simulink model "main_RI_LIEKF_GNSSOutrage"  (R2023a)
settings: Solver=FixedStepAuto  StartTime=0.0  StopTime=220  FixedStep=0.01  RelTol=1e-3
InitFcn:
  | initNavigation0612_AOA;
values from neighbouring files (symbols this model uses):
  CF_enable = 0    [initNavigation.m]
  dt = 0.01    [initNavigation.m]
  dtDelay = -0.03    [initNavigation.m]
  g0 = 9.795    [initNavigation.m]
  gam0_rad = 0/57.3    (= 0)    [initNavigation.m]
  GNSSoutragetime = 90    [initNavigation.m]
  H_sensor_type = 0    [initNavigation.m]
  KF_enable = 1    [initNavigation.m]
  P0 = diag([1*ones(3,1);0.01*ones(3,1);0.1*ones(3,1);0.001*ones(3,1);0.00001*ones(3,1)])    [initNavigation.m]
  P0_RIEKF = diag([1*ones(3,1);0.01*ones(3,1);0.1*ones(3,1);0.001*ones(3,1);0.00001*ones(3,1);      0.01*ones(3,1);[0;2;2]/57.3;[0.1;0.1;0.1]])^2    [initNavigation.m]
  pd0 = 0    [initNavigation.m]
  pe0 = 0    [initNavigation.m]
  phi0_rad = 0/57.3    (= 0)    [initNavigation.m]
  pn0 = 0    [initNavigation.m]
  psi = -178    [initNavigation.m]
  psi0_rad = 0/57.3    (= 0)    [initNavigation.m]
  state_dim = 24    [initNavigation.m]
  Time = 0:0.01:(size(traindata.AttackAngle,1) - 1)*0.01    [NNLiftCoefficientFit.m]
  vd0 = 0    [initNavigation.m]
  ve0 = 0    [initNavigation.m]
  vn0 = 0    [initNavigation.m]
undefined symbols (not defined in the file or in its folder): DiscIntNeverNeededParam, Discrete, INS_CONST, INS_EXPORT, INS_PARAM, magnitude, p, param, pInitialization, sys
libraries: simulink_extras x94, simulink x82, dspstat3 x70, sharedtransform x60, ctrlSharedLib x36, sharedTrackingLibrary x22, matrix_library x15, FMT_Model_Lib x13, deeplib x8, dspsolvers x4, vrlib x4, aerolibconvert2 x1
(part 21 of 28)

== system main_RI_LIEKF_GNSSOutrage/State estimation/RI EKF_AOA_LSTM/Error State Kalman Filter/bak/Simulink Function - State Transition Jacobian/Cal Phi1 ==
  Rbn : Inport
  vn : Inport  Port=2
  pn : Inport  Port=3
  Constant : Constant  Value=dt
  MATLAB Function1 : MATLAB Function  TreatAsAtomicUnit=on
  Reshape : Reshape  OutputDimensionality=Column vector (2-D)
  Reshape1 : Reshape  OutputDimensionality=Column vector (2-D)
  Phi : Outport
  wires:
  Constant/1 -> MATLAB Function1/4(dt)
  MATLAB Function1/1(Phi) -> Phi/1
  Rbn/1 -> MATLAB Function1/3(Rbn)
  vn/1 -> Reshape/1
  pn/1 -> Reshape1/1
  Reshape/1 -> MATLAB Function1/1(vn)
  Reshape1/1 -> MATLAB Function1/2(pn)

== system main_RI_LIEKF_GNSSOutrage/State estimation/RI EKF_AOA_LSTM/INS propogation/AOA//SA//Vwind update/Subsystem/Subsystem ==
  In1 : Inport
  v : Inport  Port=2
  Asin : Trigonometry  Operator=asin
  Math Function : Math  Operator=magnitude^2
  Product1 : Product
  Reciprocal Sqrt : Sqrt  Operator=rSqrt
  Sum of Elements : Sum  Inputs=+
  beta : Outport
  wires:
  Product1/1 -> Asin/1
  Sum of Elements/1 -> Reciprocal Sqrt/1
  Math Function/1 -> Sum of Elements/1
  Reciprocal Sqrt/1 -> Product1/1
  Asin/1 -> beta/1  "beta"
  In1/1 -> Math Function/1
  v/1 -> Product1/2

== system main_RI_LIEKF_GNSSOutrage/State estimation/RI EKF_AOA_LSTM/INS propogation/AOA//SA//Vwind update/Subsystem/Subsystem1 ==
  gyro_raw : Inport
  elevator_aileron_rudder_deg : Inport  Port=2
  accl_raw : Inport  Port=3
  TAS : Inport  Port=4
  Enable : EnablePort
  Data Type Conversion5 : DataTypeConversion  OutDataTypeStr=single  SaturateOnIntegerOverflow=off  RndMeth=Floor
  Degrees to Radians{,1..5} (6 alike) : simulink_extras/Transformations/Degrees to Radians
  LSTM predict : Subsystem
  LSTM predict1 : Subsystem
  MATLAB Function1 : MATLAB Function  TreatAsAtomicUnit=on
  MATLAB Function3 : MATLAB Function  TreatAsAtomicUnit=on
  MATLAB Function4 : MATLAB Function  Commented=on  TreatAsAtomicUnit=on
  Memory : Memory
  Memory1 : Memory
  Moving Average1 : dspstat3/Moving Average  Method=Sliding window  ForgettingFactorPort=off  SpecifyWindowLength=on  WindowLength=4  OverlapLength=3  AllowArbitraryInputLength=off  ForgettingFactor=0.9  SimulateUsing=Code generation
  Mux : Mux  Inputs=3
  Mux1 : Mux
  Radians to Degrees5 : simulink_extras/Transformations/Radians to Degrees  Commented=on
  Selector : Selector  InputPortWidth=3  IndexOptions=Index vector (dialog)  Indices=[2]  OutputSizes=1
  Selector{1..3,5} (4 alike) : Selector  InputPortWidth=3  IndexOptions=Index vector (dialog)  Indices=[1]  OutputSizes=1
  Selector4 : Selector  InputPortWidth=3  IndexOptions=Index vector (dialog)  Indices=[3]  OutputSizes=1
  Selector6 : Selector  InputPortWidth=3  IndexOptions=Index vector (dialog)  Indices=[3]  OutputSizes=1
  TAS_1 : InportShadow  Port=4
  az : InportShadow  Port=3
  elevator_aileron_rudder_deg_1 : InportShadow  Port=2
  gyro_raw_1 : InportShadow
  AOA_LSTM_rad out : Outport
  SA_LSTM_rad : Outport  Port=2
  wires:
  elevator_aileron_rudder_deg_1/1 -> Selector6/1
  TAS/1 -> Selector2/1
  gyro_raw/1 -> Selector/1
  Degrees to Radians5/1 -> SA_LSTM_rad/1
  Degrees to Radians/1 -> Mux/3
  Selector1/1 -> Degrees to Radians/1
  Memory1/1 -> MATLAB Function3/4(beta)
  MATLAB Function1/1(Cl) -> Data Type Conversion5/1
  accl_raw/1 -> MATLAB Function1/1(axyz)
  Mux/1 -> LSTM predict/1(X), MATLAB Function4/1(u)
  MATLAB Function3/1(Cy) -> Mux1/2
  Selector/1 -> Mux/1
  Selector2/1 -> MATLAB Function1/2(TAS)  "|TAS|"
  LSTM predict1/1(YPred_test_out) -> Degrees to Radians3/1, Degrees to Radians5/1  "LSTM_SA"
  Degrees to Radians3/1 -> Memory1/1
  Degrees to Radians2/1 -> Memory/1
  Degrees to Radians1/1 -> Mux1/3
  az/1 -> MATLAB Function3/1(axyz)
  Selector5/1 -> MATLAB Function3/2(TAS)  "|TAS|"
  TAS_1/1 -> Selector5/1
  LSTM predict/1(YPred_test_out) -> Moving Average1/1, Degrees to Radians4/1
  Degrees to Radians4/1 -> AOA_LSTM_rad out/1
  elevator_aileron_rudder_deg/1 -> Selector1/1
  Memory/1 -> MATLAB Function3/3(alpha), MATLAB Function1/3(alpha)
  Data Type Conversion5/1 -> Mux/2
  Selector6/1 -> Degrees to Radians1/1
  MATLAB Function4/1(CalculatedAttackAngleFiltered) -> Radians to Degrees5/1
  Mux1/1 -> LSTM predict1/1(X)
  Moving Average1/1 -> Degrees to Radians2/1  "LSTM_AOA"
  gyro_raw_1/1 -> Selector3/1, Selector4/1
  Selector3/1 -> Mux1/1
  Selector4/1 -> Mux1/4

== system main_RI_LIEKF_GNSSOutrage/State estimation/RI EKF_AOA_LSTM/INS propogation/AOA//SA//Vwind update/Subsystem/Subsystem2 ==
  In1 : Inport
  v : Inport  Port=2
  Asin : Trigonometry  Operator=asin
  Math Function : Math  Operator=magnitude^2
  Product1 : Product
  Reciprocal Sqrt : Sqrt  Operator=rSqrt
  Sum of Elements : Sum  Inputs=+
  beta : Outport
  wires:
  v/1 -> Product1/2
  In1/1 -> Math Function/1
  Asin/1 -> beta/1  "beta"
  Reciprocal Sqrt/1 -> Product1/1
  Math Function/1 -> Sum of Elements/1
  Sum of Elements/1 -> Reciprocal Sqrt/1
  Product1/1 -> Asin/1

== system main_RI_LIEKF_GNSSOutrage/State estimation/RI EKF_AOA_LSTM/INS propogation/Init_PVQ/Horizontal_attitude/Deal with zero ==
  In1 : Inport
  Add5 : Sum
  Constant1 : Constant  Value=1e-6  OutDataTypeStr=single
  Out1 : Outport
  wires:
  Add5/1 -> Out1/1
  In1/1 -> Add5/1
  Constant1/1 -> Add5/2

== system main_RI_LIEKF_GNSSOutrage/State estimation/RI EKF_AOA_LSTM/INS propogation/gyro bias compensation/error compensation/If Action Subsystem1 ==
  Action Port : ActionPort  ActionPortLabel=if(u1 == 1)
  Constant : Constant
  Data Store Write : DataStoreWrite  DataStoreName=feedback_flag_18dim_RIEKF  IndexOptions=Index vector (dialog)  Indices=1  OutputSizes=1
  wires:
  Constant/1 -> Data Store Write/1

== system main_RI_LIEKF_GNSSOutrage/State estimation/RI EKF_AOA_direct/Error State Kalman Filter/Extended Kalman Filter1/Correct1/IGG_check ==
  Pk/k_1 : Inport
  yMeas : Inport  Port=2
  X : Inport  Port=3
  R : Inport  Port=4
  Abs : Abs  Commented=on  SaturateOnIntegerOverflow=off
  Abs1 : Abs  Commented=on  SaturateOnIntegerOverflow=off
  Add : Sum  Commented=on
  Add1 : Sum  Inputs=+-
  Add2 : Sum  Commented=on
  Constant : Constant  Commented=on  Value=12
  Constant1 : Constant  Commented=on  Value=8
  Constant2 : Constant  Value=25
  Constant3 : Constant  Commented=on  Value=eps
  Constant4 : Constant  Commented=on  Value=15
  Constant6 : Constant  Value=[zeros(6,3),eye(6),zeros(6,6)]  OutDataTypeStr=single
  Divide : Product  Commented=on  Inputs=*/
  Extract Diagonal1 : matrix_library/Extract Diagonal  Commented=on
  MATLAB Function : MATLAB Function  Commented=on  TreatAsAtomicUnit=on
  Product : Product  Inputs=3  Multiplication=Matrix(*)
  Product1 : Product  Multiplication=Matrix(*)
  Product2 : Product
  Scope : Scope  Commented=on
  Sqrt1 : Sqrt  Commented=on
  Transpose : Math  Operator=transpose
  yMeas1 : InportShadow  Port=2
  yMeas_out : Outport
  w : Outport  Port=2
  inno : Outport  Port=3
  wires:
  Constant2/1 -> MATLAB Function/5(zk1)
  Constant/1 -> MATLAB Function/4(zk0)
  Constant4/1 -> MATLAB Function/3(k1)
  Constant1/1 -> MATLAB Function/2(k0)
  yMeas1/1 -> Product2/2
  Constant3/1 -> Add2/2
  Add2/1 -> Divide/2
  Abs1/1 -> Sqrt1/1
  Abs/1 -> MATLAB Function/1(err)
  Sqrt1/1 -> Add2/1
  Add1/1 -> Divide/1, inno/1
  Extract Diagonal1/1 -> Abs1/1
  MATLAB Function/1(w) -> Product2/1, w/1
  Divide/1 -> Scope/1, Abs/1
  Add/1 -> Extract Diagonal1/1  "S"
  Product2/1 -> yMeas_out/1
  Product1/1 -> Add1/2
  X/1 -> Product1/2
  Constant6/1 -> Transpose/1, Product/1, Product1/1
  yMeas/1 -> Add1/1
  Pk/k_1/1 -> Product/2
  R/1 -> Add/2
  Transpose/1 -> Product/3
  Product/1 -> Add/1

== system main_RI_LIEKF_GNSSOutrage/State estimation/RI EKF_AOA_direct/Error State Kalman Filter/Extended Kalman Filter1/Predict/If Action Subsystem ==
  Action Port : ActionPort
  Constant : Constant  Value=0
  Data Store Read : DataStoreRead  DataStoreName=x  IndexOptions=Index vector (dialog)  Indices=1  OutputSizes=1
  Data Store Write : DataStoreWrite  DataStoreName=x  IndexOptions=Index vector (dialog)  Indices=1  OutputSizes=1
  Data Store Write1 : DataStoreWrite  DataStoreName=feedback_flag_18dim  IndexOptions=Index vector (dialog)  Indices=1  OutputSizes=1
  Mux : Mux  Inputs=2
  Selector : Selector  InputPortWidth=18  IndexOptions=Index vector (dialog)  Indices=[16 17 18]  OutputSizes=1
  Zero : Constant  Value=zeros(15,1)  OutDataTypeStr=Inherit: Inherit via back propagation
  wires:
  Constant/1 -> Data Store Write1/1
  Data Store Read/1 -> Selector/1
  Zero/1 -> Mux/1
  Selector/1 -> Mux/2
  Mux/1 -> Data Store Write/1

== system main_RI_LIEKF_GNSSOutrage/State estimation/RI EKF_AOA_direct/Error State Kalman Filter/bak/Simulink Function - State Transition Jacobian/Cal Phi1 ==
  Rbn : Inport
  vn : Inport  Port=2
  pn : Inport  Port=3
  Constant : Constant  Value=dt
  MATLAB Function1 : MATLAB Function  TreatAsAtomicUnit=on
  Reshape : Reshape  OutputDimensionality=Column vector (2-D)
  Reshape1 : Reshape  OutputDimensionality=Column vector (2-D)
  Phi : Outport
  wires:
  Reshape1/1 -> MATLAB Function1/2(pn)
  Reshape/1 -> MATLAB Function1/1(vn)
  pn/1 -> Reshape1/1
  vn/1 -> Reshape/1
  Rbn/1 -> MATLAB Function1/3(Rbn)
  MATLAB Function1/1(Phi) -> Phi/1
  Constant/1 -> MATLAB Function1/4(dt)

== system main_RI_LIEKF_GNSSOutrage/State estimation/RI EKF_AOA_direct/INS propogation/AOA//SA//Vwind update/Subsystem/Subsystem ==
  In1 : Inport
  v : Inport  Port=2
  Asin : Trigonometry  Operator=asin
  Math Function : Math  Operator=magnitude^2
  Product1 : Product
  Reciprocal Sqrt : Sqrt  Operator=rSqrt
  Sum of Elements : Sum  Inputs=+
  beta : Outport
  wires:
  v/1 -> Product1/2
  In1/1 -> Math Function/1
  Asin/1 -> beta/1  "beta"
  Reciprocal Sqrt/1 -> Product1/1
  Math Function/1 -> Sum of Elements/1
  Sum of Elements/1 -> Reciprocal Sqrt/1
  Product1/1 -> Asin/1

== system main_RI_LIEKF_GNSSOutrage/State estimation/RI EKF_AOA_direct/INS propogation/AOA//SA//Vwind update/Subsystem/Subsystem1 ==
  gyro_raw : Inport
  elevator_aileron_rudder_deg : Inport  Port=2
  accl_raw : Inport  Port=3
  TAS : Inport  Port=4
  Enable : EnablePort
  Data Type Conversion5 : DataTypeConversion  OutDataTypeStr=single  SaturateOnIntegerOverflow=off  RndMeth=Floor
  Degrees to Radians{,1..5} (6 alike) : simulink_extras/Transformations/Degrees to Radians
  LSTM predict : Subsystem
  LSTM predict1 : Subsystem
  MATLAB Function1 : MATLAB Function  TreatAsAtomicUnit=on
  MATLAB Function3 : MATLAB Function  TreatAsAtomicUnit=on
  MATLAB Function4 : MATLAB Function  Commented=on  TreatAsAtomicUnit=on
  Memory : Memory
  Memory1 : Memory
  Moving Average : dspstat3/Moving Average  Method=Sliding window  ForgettingFactorPort=off  SpecifyWindowLength=on  WindowLength=4  OverlapLength=3  AllowArbitraryInputLength=off  ForgettingFactor=0.9  SimulateUsing=Code generation
  Moving Average1 : dspstat3/Moving Average  Method=Sliding window  ForgettingFactorPort=off  SpecifyWindowLength=on  WindowLength=4  OverlapLength=3  AllowArbitraryInputLength=off  ForgettingFactor=0.9  SimulateUsing=Code generation
  Mux : Mux  Inputs=3
  Mux1 : Mux
  Radians to Degrees5 : simulink_extras/Transformations/Radians to Degrees  Commented=on
  Selector : Selector  InputPortWidth=3  IndexOptions=Index vector (dialog)  Indices=[2]  OutputSizes=1
  Selector{1..3,5} (4 alike) : Selector  InputPortWidth=3  IndexOptions=Index vector (dialog)  Indices=[1]  OutputSizes=1
  Selector4 : Selector  InputPortWidth=3  IndexOptions=Index vector (dialog)  Indices=[3]  OutputSizes=1
  Selector6 : Selector  InputPortWidth=3  IndexOptions=Index vector (dialog)  Indices=[3]  OutputSizes=1
  TAS_1 : InportShadow  Port=4
  az : InportShadow  Port=3
  elevator_aileron_rudder_deg_1 : InportShadow  Port=2
  gyro_raw_1 : InportShadow
  AOA_LSTM_rad out : Outport
  SA_LSTM_rad : Outport  Port=2
  wires:
  Moving Average1/1 -> Degrees to Radians2/1  "LSTM_AOA"
  Selector4/1 -> Mux1/4
  Mux1/1 -> LSTM predict1/1(X)
  MATLAB Function4/1(CalculatedAttackAngleFiltered) -> Radians to Degrees5/1
  Selector6/1 -> Degrees to Radians1/1
  Data Type Conversion5/1 -> Mux/2
  Selector3/1 -> Mux1/1
  Memory/1 -> MATLAB Function1/3(alpha), MATLAB Function3/3(alpha)
  elevator_aileron_rudder_deg/1 -> Selector1/1
  LSTM predict1/1(YPred_test_out) -> Moving Average/1, Degrees to Radians5/1
  Degrees to Radians4/1 -> AOA_LSTM_rad out/1
  LSTM predict/1(YPred_test_out) -> Degrees to Radians4/1, Moving Average1/1
  TAS_1/1 -> Selector5/1
  Selector5/1 -> MATLAB Function3/2(TAS)  "|TAS|"
  az/1 -> MATLAB Function3/1(axyz)
  Degrees to Radians1/1 -> Mux1/3
  Degrees to Radians2/1 -> Memory/1
  Degrees to Radians3/1 -> Memory1/1
  Moving Average/1 -> Degrees to Radians3/1  "LSTM_SA"
  Selector2/1 -> MATLAB Function1/2(TAS)  "|TAS|"
  Selector/1 -> Mux/1
  MATLAB Function3/1(Cy) -> Mux1/2
  Mux/1 -> MATLAB Function4/1(u), LSTM predict/1(X)
  gyro_raw_1/1 -> Selector4/1, Selector3/1
  accl_raw/1 -> MATLAB Function1/1(axyz)
  MATLAB Function1/1(Cl) -> Data Type Conversion5/1
  Memory1/1 -> MATLAB Function3/4(beta)
  Selector1/1 -> Degrees to Radians/1
  Degrees to Radians/1 -> Mux/3
  Degrees to Radians5/1 -> SA_LSTM_rad/1
  gyro_raw/1 -> Selector/1
  TAS/1 -> Selector2/1
  elevator_aileron_rudder_deg_1/1 -> Selector6/1

== system main_RI_LIEKF_GNSSOutrage/State estimation/RI EKF_AOA_direct/INS propogation/AOA//SA//Vwind update/Subsystem/Subsystem3 ==
  RIEKF_att_Deg : Inport
  vel_NED : Inport  Port=2
  psi_Deg : Inport  Port=3
  Enable : EnablePort
  Add1 : Sum  Inputs=+-
  Add2 : Sum  Inputs=+-
  Asin1 : Trigonometry  Operator=asin
  Atan2 : Trigonometry  Operator=atan2
  Divide1 : Product  Inputs=*/
  Fcn : Fcn  Expr=sqrt(u(1)^2+u(2)^2+u(3)^2)
  Gain : Gain  Gain=-1
  Radians to Degrees{1..4} (4 alike) : simulink_extras/Transformations/Radians to Degrees
  Selector1 : Selector  InputPortWidth=3  IndexOptions=Index vector (dialog)  Indices=[2]  OutputSizes=1
  Selector2 : Selector  InputPortWidth=3  IndexOptions=Index vector (dialog)  Indices=[3]  OutputSizes=1
  Selector3 : Selector  InputPortWidth=3  IndexOptions=Index vector (dialog)  Indices=[1]  OutputSizes=1
  AOA_direct_Deg : Outport
  SA_direct_Deg : Outport  Port=2
  wires:
  RIEKF_att_Deg/1 -> Radians to Degrees2/1
  Radians to Degrees3/1 -> Add1/2  "theta"
  Divide1/1 -> Asin1/1
  Selector2/1 -> Gain/1
  vel_NED/1 -> Selector3/1, Selector1/1, Fcn/1, Selector2/1
  Asin1/1 -> Radians to Degrees3/1
  Fcn/1 -> Divide1/2
  Gain/1 -> Divide1/1
  Add1/1 -> AOA_direct_Deg/1  "AOA_direct"
  Selector1/1 -> Atan2/1
  Selector3/1 -> Atan2/2
  Atan2/1 -> Radians to Degrees1/1
  psi_Deg/1 -> Radians to Degrees4/1
  Radians to Degrees1/1 -> Add2/2  "theta"
  Add2/1 -> SA_direct_Deg/1  "SA_direct"
  Radians to Degrees2/1 -> Add1/1  "theta"
  Radians to Degrees4/1 -> Add2/1  "theta"

== system main_RI_LIEKF_GNSSOutrage/State estimation/RI EKF_AOA_direct/INS propogation/AOA//SA//Vwind update/Subsystem/Subsystem4 ==
  vel_NED : Inport
  Compare To Constant : simulink/Logic and Bit Operations/Compare To Constant  relop=>=  const=10  OutDataTypeStr=boolean
  Math Function : Math  Operator=magnitude^2
  Sqrt : Sqrt
  Sum of Elements : Sum  Inputs=+
  AOA_Estimation_flag : Outport
  wires:
  Sum of Elements/1 -> Sqrt/1
  Sqrt/1 -> Compare To Constant/1
  Compare To Constant/1 -> AOA_Estimation_flag/1
  Math Function/1 -> Sum of Elements/1
  vel_NED/1 -> Math Function/1

== system main_RI_LIEKF_GNSSOutrage/State estimation/RI EKF_AOA_direct/INS propogation/Init_PVQ/Horizontal_attitude/Deal with zero ==
  In1 : Inport
  Add5 : Sum
  Constant1 : Constant  Value=1e-6  OutDataTypeStr=single
  Out1 : Outport
  wires:
  Constant1/1 -> Add5/2
  In1/1 -> Add5/1
  Add5/1 -> Out1/1

== system main_RI_LIEKF_GNSSOutrage/State estimation/RI EKF_AOA_direct/INS propogation/gyro bias compensation/error compensation/If Action Subsystem1 ==
  Action Port : ActionPort  ActionPortLabel=if(u1 == 1)
  Constant : Constant
  Data Store Write : DataStoreWrite  DataStoreName=feedback_flag_18dim_RIEKF  IndexOptions=Index vector (dialog)  Indices=1  OutputSizes=1
  wires:
  Constant/1 -> Data Store Write/1

== system main_RI_LIEKF_GNSSOutrage/State estimation/RI EKF_AOA_ref/Error State Kalman Filter/Extended Kalman Filter1/Correct1/IGG_check ==
  Pk/k_1 : Inport
  yMeas : Inport  Port=2
  X : Inport  Port=3
  R : Inport  Port=4
  Abs : Abs  Commented=on  SaturateOnIntegerOverflow=off
  Abs1 : Abs  Commented=on  SaturateOnIntegerOverflow=off
  Add : Sum  Commented=on
  Add1 : Sum  Inputs=+-
  Add2 : Sum  Commented=on
  Constant : Constant  Commented=on  Value=12
  Constant1 : Constant  Commented=on  Value=8
  Constant2 : Constant  Value=25
  Constant3 : Constant  Commented=on  Value=eps
  Constant4 : Constant  Commented=on  Value=15
  Constant6 : Constant  Value=[zeros(6,3),eye(6),zeros(6,6)]  OutDataTypeStr=single
  Divide : Product  Commented=on  Inputs=*/
  Extract Diagonal1 : matrix_library/Extract Diagonal  Commented=on
  MATLAB Function : MATLAB Function  Commented=on  TreatAsAtomicUnit=on
  Product : Product  Inputs=3  Multiplication=Matrix(*)
  Product1 : Product  Multiplication=Matrix(*)
  Product2 : Product
  Scope : Scope  Commented=on
  Sqrt1 : Sqrt  Commented=on
  Transpose : Math  Operator=transpose
  yMeas1 : InportShadow  Port=2
  yMeas_out : Outport
  w : Outport  Port=2
  inno : Outport  Port=3
  wires:
  Constant2/1 -> MATLAB Function/5(zk1)
  Constant/1 -> MATLAB Function/4(zk0)
  Constant4/1 -> MATLAB Function/3(k1)
  Constant1/1 -> MATLAB Function/2(k0)
  yMeas1/1 -> Product2/2
  Constant3/1 -> Add2/2
  Add2/1 -> Divide/2
  Abs1/1 -> Sqrt1/1
  Abs/1 -> MATLAB Function/1(err)
  Sqrt1/1 -> Add2/1
  Add1/1 -> Divide/1, inno/1
  Extract Diagonal1/1 -> Abs1/1
  MATLAB Function/1(w) -> Product2/1, w/1
  Divide/1 -> Scope/1, Abs/1
  Add/1 -> Extract Diagonal1/1  "S"
  Product2/1 -> yMeas_out/1
  Product1/1 -> Add1/2
  X/1 -> Product1/2
  Constant6/1 -> Transpose/1, Product/1, Product1/1
  yMeas/1 -> Add1/1
  Pk/k_1/1 -> Product/2
  R/1 -> Add/2
  Transpose/1 -> Product/3
  Product/1 -> Add/1

== system main_RI_LIEKF_GNSSOutrage/State estimation/RI EKF_AOA_ref/Error State Kalman Filter/Extended Kalman Filter1/Predict/If Action Subsystem ==
  Action Port : ActionPort
  Constant : Constant  Value=0
  Data Store Read : DataStoreRead  DataStoreName=x  IndexOptions=Index vector (dialog)  Indices=1  OutputSizes=1
  Data Store Write : DataStoreWrite  DataStoreName=x  IndexOptions=Index vector (dialog)  Indices=1  OutputSizes=1
  Data Store Write1 : DataStoreWrite  DataStoreName=feedback_flag_18dim  IndexOptions=Index vector (dialog)  Indices=1  OutputSizes=1
  Mux : Mux  Inputs=2
  Selector : Selector  InputPortWidth=18  IndexOptions=Index vector (dialog)  Indices=[16 17 18]  OutputSizes=1
  Zero : Constant  Value=zeros(15,1)  OutDataTypeStr=Inherit: Inherit via back propagation
  wires:
  Constant/1 -> Data Store Write1/1
  Data Store Read/1 -> Selector/1
  Zero/1 -> Mux/1
  Selector/1 -> Mux/2
  Mux/1 -> Data Store Write/1

== system main_RI_LIEKF_GNSSOutrage/State estimation/RI EKF_AOA_ref/Error State Kalman Filter/bak/Simulink Function - State Transition Jacobian/Cal Phi1 ==
  Rbn : Inport
  vn : Inport  Port=2
  pn : Inport  Port=3
  Constant : Constant  Value=dt
  MATLAB Function1 : MATLAB Function  TreatAsAtomicUnit=on
  Reshape : Reshape  OutputDimensionality=Column vector (2-D)
  Reshape1 : Reshape  OutputDimensionality=Column vector (2-D)
  Phi : Outport
  wires:
  Reshape1/1 -> MATLAB Function1/2(pn)
  Reshape/1 -> MATLAB Function1/1(vn)
  pn/1 -> Reshape1/1
  vn/1 -> Reshape/1
  Rbn/1 -> MATLAB Function1/3(Rbn)
  MATLAB Function1/1(Phi) -> Phi/1
  Constant/1 -> MATLAB Function1/4(dt)

== system main_RI_LIEKF_GNSSOutrage/State estimation/RI EKF_AOA_ref/INS propogation/AOA//SA//Vwind update/Subsystem/Subsystem ==
  In1 : Inport
  v : Inport  Port=2
  Asin : Trigonometry  Operator=asin
  Math Function : Math  Operator=magnitude^2
  Product1 : Product
  Reciprocal Sqrt : Sqrt  Operator=rSqrt
  Sum of Elements : Sum  Inputs=+
  beta : Outport
  wires:
  v/1 -> Product1/2
  In1/1 -> Math Function/1
  Asin/1 -> beta/1  "beta"
  Reciprocal Sqrt/1 -> Product1/1
  Math Function/1 -> Sum of Elements/1
  Sum of Elements/1 -> Reciprocal Sqrt/1
  Product1/1 -> Asin/1

== system main_RI_LIEKF_GNSSOutrage/State estimation/RI EKF_AOA_ref/INS propogation/AOA//SA//Vwind update/Subsystem/Subsystem1 ==
  gyro_raw : Inport
  elevator_aileron_rudder_deg : Inport  Port=2
  accl_raw : Inport  Port=3
  TAS : Inport  Port=4
  Enable : EnablePort
  Data Type Conversion5 : DataTypeConversion  OutDataTypeStr=single  SaturateOnIntegerOverflow=off  RndMeth=Floor
  Degrees to Radians{,1..5} (6 alike) : simulink_extras/Transformations/Degrees to Radians
  LSTM predict : Subsystem
  LSTM predict1 : Subsystem
  MATLAB Function1 : MATLAB Function  TreatAsAtomicUnit=on
  MATLAB Function3 : MATLAB Function  TreatAsAtomicUnit=on
  MATLAB Function4 : MATLAB Function  Commented=on  TreatAsAtomicUnit=on
  Memory : Memory
  Memory1 : Memory
  Moving Average1 : dspstat3/Moving Average  Method=Sliding window  ForgettingFactorPort=off  SpecifyWindowLength=on  WindowLength=4  OverlapLength=3  AllowArbitraryInputLength=off  ForgettingFactor=0.9  SimulateUsing=Code generation
  Mux : Mux  Inputs=3
  Mux1 : Mux
  Radians to Degrees5 : simulink_extras/Transformations/Radians to Degrees  Commented=on
  Selector : Selector  InputPortWidth=3  IndexOptions=Index vector (dialog)  Indices=[2]  OutputSizes=1
  Selector{1..3,5} (4 alike) : Selector  InputPortWidth=3  IndexOptions=Index vector (dialog)  Indices=[1]  OutputSizes=1
  Selector4 : Selector  InputPortWidth=3  IndexOptions=Index vector (dialog)  Indices=[3]  OutputSizes=1
  Selector6 : Selector  InputPortWidth=3  IndexOptions=Index vector (dialog)  Indices=[3]  OutputSizes=1
  TAS_1 : InportShadow  Port=4
  az : InportShadow  Port=3
  elevator_aileron_rudder_deg_1 : InportShadow  Port=2
  gyro_raw_1 : InportShadow
  AOA_LSTM_rad out : Outport
  SA_LSTM_rad : Outport  Port=2
  wires:
  Selector4/1 -> Mux1/4
  Selector3/1 -> Mux1/1
  gyro_raw_1/1 -> Selector4/1, Selector3/1
  Moving Average1/1 -> Degrees to Radians2/1  "LSTM_AOA"
  Mux1/1 -> LSTM predict1/1(X)
  MATLAB Function4/1(CalculatedAttackAngleFiltered) -> Radians to Degrees5/1
  Selector6/1 -> Degrees to Radians1/1
  Data Type Conversion5/1 -> Mux/2
  Memory/1 -> MATLAB Function1/3(alpha), MATLAB Function3/3(alpha)
  elevator_aileron_rudder_deg/1 -> Selector1/1
  Degrees to Radians4/1 -> AOA_LSTM_rad out/1
  LSTM predict/1(YPred_test_out) -> Degrees to Radians4/1, Moving Average1/1
  TAS_1/1 -> Selector5/1
  Selector5/1 -> MATLAB Function3/2(TAS)  "|TAS|"
  az/1 -> MATLAB Function3/1(axyz)
  Degrees to Radians1/1 -> Mux1/3
  Degrees to Radians2/1 -> Memory/1
  Degrees to Radians3/1 -> Memory1/1
  LSTM predict1/1(YPred_test_out) -> Degrees to Radians5/1, Degrees to Radians3/1  "LSTM_SA"
  Selector2/1 -> MATLAB Function1/2(TAS)  "|TAS|"
  Selector/1 -> Mux/1
  MATLAB Function3/1(Cy) -> Mux1/2
  Mux/1 -> MATLAB Function4/1(u), LSTM predict/1(X)
  accl_raw/1 -> MATLAB Function1/1(axyz)
  MATLAB Function1/1(Cl) -> Data Type Conversion5/1
  Memory1/1 -> MATLAB Function3/4(beta)
  Selector1/1 -> Degrees to Radians/1
  Degrees to Radians/1 -> Mux/3
  Degrees to Radians5/1 -> SA_LSTM_rad/1
  gyro_raw/1 -> Selector/1
  TAS/1 -> Selector2/1
  elevator_aileron_rudder_deg_1/1 -> Selector6/1

== system main_RI_LIEKF_GNSSOutrage/State estimation/RI EKF_AOA_ref/INS propogation/AOA//SA//Vwind update/Subsystem/Subsystem2 ==
  In1 : Inport
  v : Inport  Port=2
  Asin : Trigonometry  Operator=asin
  Math Function : Math  Operator=magnitude^2
  Product1 : Product
  Reciprocal Sqrt : Sqrt  Operator=rSqrt
  Sum of Elements : Sum  Inputs=+
  beta : Outport
  wires:
  Product1/1 -> Asin/1
  Sum of Elements/1 -> Reciprocal Sqrt/1
  Math Function/1 -> Sum of Elements/1
  Reciprocal Sqrt/1 -> Product1/1
  Asin/1 -> beta/1  "beta"
  In1/1 -> Math Function/1
  v/1 -> Product1/2

== system main_RI_LIEKF_GNSSOutrage/State estimation/RI EKF_AOA_ref/INS propogation/Init_PVQ/Horizontal_attitude/Deal with zero ==
  In1 : Inport
  Add5 : Sum
  Constant1 : Constant  Value=1e-6  OutDataTypeStr=single
  Out1 : Outport
  wires:
  Constant1/1 -> Add5/2
  In1/1 -> Add5/1
  Add5/1 -> Out1/1

== system main_RI_LIEKF_GNSSOutrage/State estimation/RI EKF_AOA_ref/INS propogation/gyro bias compensation/error compensation/If Action Subsystem1 ==
  Action Port : ActionPort  ActionPortLabel=if(u1 == 1)
  Constant : Constant
  Data Store Write : DataStoreWrite  DataStoreName=feedback_flag_18dim_RIEKF  IndexOptions=Index vector (dialog)  Indices=1  OutputSizes=1
  wires:
  Constant/1 -> Data Store Write/1

== system main_RI_LIEKF_GNSSOutrage/State estimation/RI UKF/Error State Kalman Filter/bak/Simulink Function - State Transition Jacobian/Cal Phi1 ==
  Rbn : Inport
  vn : Inport  Port=2
  pn : Inport  Port=3
  Constant : Constant  Value=dt
  MATLAB Function1 : MATLAB Function  TreatAsAtomicUnit=on
  Reshape : Reshape  OutputDimensionality=Column vector (2-D)
  Reshape1 : Reshape  OutputDimensionality=Column vector (2-D)
  Phi : Outport
  wires:
  Constant/1 -> MATLAB Function1/4(dt)
  MATLAB Function1/1(Phi) -> Phi/1
  Rbn/1 -> MATLAB Function1/3(Rbn)
  vn/1 -> Reshape/1
  pn/1 -> Reshape1/1
  Reshape/1 -> MATLAB Function1/1(vn)
  Reshape1/1 -> MATLAB Function1/2(pn)

== system main_RI_LIEKF_GNSSOutrage/State estimation/RI UKF/INS propogation/AOA//SA//Vwind update/Subsystem/Subsystem ==
  In1 : Inport
  v : Inport  Port=2
  Asin : Trigonometry  Operator=asin
  Math Function : Math  Operator=magnitude^2
  Product1 : Product
  Reciprocal Sqrt : Sqrt  Operator=rSqrt
  Sum of Elements : Sum  Inputs=+
  beta : Outport
  wires:
  Product1/1 -> Asin/1
  Sum of Elements/1 -> Reciprocal Sqrt/1
  Math Function/1 -> Sum of Elements/1
  Reciprocal Sqrt/1 -> Product1/1
  Asin/1 -> beta/1  "beta"
  In1/1 -> Math Function/1
  v/1 -> Product1/2

== system main_RI_LIEKF_GNSSOutrage/State estimation/RI UKF/INS propogation/Init_PVQ/Horizontal_attitude/Deal with zero ==
  In1 : Inport
  Add5 : Sum
  Constant1 : Constant  Value=1e-6  OutDataTypeStr=single
  Out1 : Outport
  wires:
  Add5/1 -> Out1/1
  In1/1 -> Add5/1
  Constant1/1 -> Add5/2

== system main_RI_LIEKF_GNSSOutrage/State estimation/RI UKF/INS propogation/gyro bias compensation/error compensation/If Action Subsystem1 ==
  Action Port : ActionPort  ActionPortLabel=if(u1 == 1)
  Constant : Constant
  Data Store Write : DataStoreWrite  DataStoreName=feedback_flag_18dim  IndexOptions=Index vector (dialog)  Indices=1  OutputSizes=1
  wires:
  Constant/1 -> Data Store Write/1

== system main_RI_LIEKF_GNSSOutrage/State estimation/bak1/Error State Kalman Filter/Extended Kalman Filter1/Correct1/IGG_check ==
  Pk/k_1 : Inport
  yMeas : Inport  Port=2
  X : Inport  Port=3
  R : Inport  Port=4
  Abs : Abs  SaturateOnIntegerOverflow=off
  Abs1 : Abs  SaturateOnIntegerOverflow=off
  Add : Sum
  Add1 : Sum  Inputs=+-
  Add2 : Sum
  Constant : Constant  Value=12
  Constant1 : Constant  Value=8
  Constant2 : Constant  Value=25
  Constant3 : Constant  Value=eps
  Constant4 : Constant  Value=15
  Constant6 : Constant  Value=[eye(3),zeros(3,15)]  OutDataTypeStr=single
  Divide : Product  Inputs=*/
  Extract Diagonal1 : matrix_library/Extract Diagonal
  MATLAB Function : MATLAB Function  TreatAsAtomicUnit=on
  Product : Product  Inputs=3  Multiplication=Matrix(*)
  Product1 : Product  Multiplication=Matrix(*)
  Product2 : Product
  Scope : Scope
  Sqrt1 : Sqrt
  Transpose : Math  Operator=transpose
  yMeas1 : InportShadow  Port=2
  yMeas_out : Outport
  w : Outport  Port=2
  wires:
  Constant2/1 -> MATLAB Function/5(zk1)
  Constant/1 -> MATLAB Function/4(zk0)
  Constant4/1 -> MATLAB Function/3(k1)
  Constant1/1 -> MATLAB Function/2(k0)
  yMeas1/1 -> Product2/2
  Constant3/1 -> Add2/2
  Add2/1 -> Divide/2
  Abs1/1 -> Sqrt1/1
  Abs/1 -> MATLAB Function/1(err)
  Sqrt1/1 -> Add2/1
  Add1/1 -> Divide/1
  Extract Diagonal1/1 -> Abs1/1
  MATLAB Function/1(w) -> Product2/1, w/1
  Divide/1 -> Scope/1, Abs/1
  Add/1 -> Extract Diagonal1/1  "S"
  Product2/1 -> yMeas_out/1
  Product1/1 -> Add1/2
  X/1 -> Product1/2
  Constant6/1 -> Transpose/1, Product/1, Product1/1
  yMeas/1 -> Add1/1
  Pk/k_1/1 -> Product/2
  R/1 -> Add/2
  Transpose/1 -> Product/3
  Product/1 -> Add/1

== system main_RI_LIEKF_GNSSOutrage/State estimation/bak1/Error State Kalman Filter/Extended Kalman Filter1/Predict/If Action Subsystem ==
  Action Port : ActionPort
  Constant : Constant  Value=0
  Data Store Read : DataStoreRead  DataStoreName=x  IndexOptions=Index vector (dialog)  Indices=1  OutputSizes=1
  Data Store Write : DataStoreWrite  DataStoreName=x  IndexOptions=Index vector (dialog)  Indices=1  OutputSizes=1
  Data Store Write1 : DataStoreWrite  DataStoreName=feedback_flag_18dim  IndexOptions=Index vector (dialog)  Indices=1  OutputSizes=1
  Mux : Mux  Inputs=2
  Selector : Selector  InputPortWidth=18  IndexOptions=Index vector (dialog)  Indices=[16 17 18]  OutputSizes=1
  Zero : Constant  Value=zeros(15,1)  OutDataTypeStr=Inherit: Inherit via back propagation
  wires:
  Constant/1 -> Data Store Write1/1
  Data Store Read/1 -> Selector/1
  Zero/1 -> Mux/1
  Selector/1 -> Mux/2
  Mux/1 -> Data Store Write/1

== system main_RI_LIEKF_GNSSOutrage/State estimation/bak1/INS propogation/Init_PVQ/Horizontal_attitude/Deal with zero ==
  In1 : Inport
  Add5 : Sum
  Constant1 : Constant  Value=1e-6  OutDataTypeStr=single
  Out1 : Outport
  wires:
  Constant1/1 -> Add5/2
  In1/1 -> Add5/1
  Add5/1 -> Out1/1

== system main_RI_LIEKF_GNSSOutrage/State estimation/bak1/INS propogation/gyro bias compensation/error compensation/If Action Subsystem1 ==
  Action Port : ActionPort
  Constant : Constant
  Data Store Write : DataStoreWrite  DataStoreName=feedback_flag_18dim  IndexOptions=Index vector (dialog)  Indices=1  OutputSizes=1
  wires:
  Constant/1 -> Data Store Write/1

== system main_RI_LIEKF_GNSSOutrage/State estimation/distribute CF/AHRS/AHRS Complementary filter/Complementary Filter/Cross-product ==
  vactor_A : Inport
  vactor_B : Inport  Port=2
  Bus Creator : BusCreator  Inputs=6
  Demux : Demux  Outputs=3
  Demux1 : Demux  Outputs=3
  Fcn : Fcn  Expr=u(2)*u(6)-u(3)*u(5)
  Fcn1 : Fcn  Expr=u(3)*u(4)-u(1)*u(6)
  Fcn2 : Fcn  Expr=u(1)*u(5)-u(2)*u(4)
  Mux2 : Mux  Inputs=3
  vactor_error_A&B : Outport
  wires:
  Demux/1 -> Bus Creator/1
  Demux/2 -> Bus Creator/2
  Demux/3 -> Bus Creator/3
  Demux1/1 -> Bus Creator/4
  Demux1/2 -> Bus Creator/5
  Demux1/3 -> Bus Creator/6
  Bus Creator/1 -> Fcn2/1, Fcn1/1, Fcn/1
  Fcn/1 -> Mux2/1
  Fcn1/1 -> Mux2/2
  Fcn2/1 -> Mux2/3
  vactor_A/1 -> Demux/1
  Mux2/1 -> vactor_error_A&B/1
  vactor_B/1 -> Demux1/1

== system main_RI_LIEKF_GNSSOutrage/State estimation/distribute CF/AHRS/AHRS Complementary filter/Complementary Filter/Normalized ==
  fb : Inport
  Divide : Product  Inputs=*/
  Math Function : Math  Operator=magnitude^2  SignedPower=on
  Sqrt : Sqrt
  Sum of Elements : Sum  Inputs=+
  fb/g : Outport
  wires:
  Math Function/1 -> Sum of Elements/1
  Divide/1 -> fb/g/1
  Sum of Elements/1 -> Sqrt/1
  fb/1 -> Divide/1, Math Function/1
  Sqrt/1 -> Divide/2

== system main_RI_LIEKF_GNSSOutrage/State estimation/distribute CF/AHRS/AHRS Complementary filter/Complementary Filter/Normalized1 ==
  fb_estimatedValue : Inport
  Divide : Product  Inputs=*/
  Math Function : Math  Operator=magnitude^2  SignedPower=on
  Sqrt : Sqrt
  Sum of Elements : Sum  Inputs=+
  fb_estimatedValue_Normalized : Outport
  wires:
  Math Function/1 -> Sum of Elements/1
  Divide/1 -> fb_estimatedValue_Normalized/1
  Sum of Elements/1 -> Sqrt/1
  fb_estimatedValue/1 -> Divide/1, Math Function/1
  Sqrt/1 -> Divide/2

== system main_RI_LIEKF_GNSSOutrage/State estimation/distribute CF/AHRS/AHRS Complementary filter/MagnHeadingCorrect/Subsystem6 ==
  m : Inport
  Add : Sum  Inputs=3
  Demux : Demux  Outputs=3
  Divide : Product  Inputs=*/
  Dot Product : DotProduct  OutDataTypeStr=Inherit: Inherit via internal rule
  Dot Product1 : DotProduct  OutDataTypeStr=Inherit: Inherit via internal rule
  Dot Product2 : DotProduct  OutDataTypeStr=Inherit: Inherit via internal rule
  Sqrt : Sqrt
  Switch : Switch  Criteria=u2 > Threshold  SaturateOnIntegerOverflow=off  InputSameDT=off
  z : Constant  Value=zeros(3,1)  OutDataTypeStr=single
  m/|m| : Outport
  wires:
  Switch/1 -> m/|m|/1
  z/1 -> Switch/3
  Sqrt/1 -> Divide/2, Switch/2
  Dot Product2/1 -> Add/3
  Dot Product/1 -> Add/1
  Dot Product1/1 -> Add/2
  Demux/1 -> Dot Product/2, Dot Product/1
  m/1 -> Demux/1, Divide/1
  Add/1 -> Sqrt/1
  Divide/1 -> Switch/1
  Demux/3 -> Dot Product2/1, Dot Product2/2
  Demux/2 -> Dot Product1/1, Dot Product1/2

== system main_RI_LIEKF_GNSSOutrage/State estimation/distribute CF/AHRS/AHRS Complementary filter/MagnHeadingCorrect/chacheng6 ==
  In1 : Inport
  In2 : Inport  Port=2
  Bus Creator : BusCreator  Inputs=6
  Demux : Demux  Outputs=3
  Demux1 : Demux  Outputs=3
  Fcn : Fcn  Expr=u(2)*u(6)-u(3)*u(5)
  Fcn1 : Fcn  Expr=u(3)*u(4)-u(1)*u(6)
  Fcn2 : Fcn  Expr=u(1)*u(5)-u(2)*u(4)
  Mux2 : Mux  Inputs=3
  Out1 : Outport
  wires:
  In2/1 -> Demux1/1
  Mux2/1 -> Out1/1
  In1/1 -> Demux/1
  Fcn2/1 -> Mux2/3
  Fcn1/1 -> Mux2/2
  Fcn/1 -> Mux2/1
  Bus Creator/1 -> Fcn2/1, Fcn1/1, Fcn/1
  Demux1/3 -> Bus Creator/6
  Demux1/2 -> Bus Creator/5
  Demux1/1 -> Bus Creator/4
  Demux/3 -> Bus Creator/3
  Demux/2 -> Bus Creator/2
  Demux/1 -> Bus Creator/1

== system main_RI_LIEKF_GNSSOutrage/State estimation/distribute CF/AHRS/AHRS Complementary filter/manoeuvrable check/manoeuvrable check ==
  fn : Inport
  eular : Inport  Port=2
  manoeuvrable check : MATLAB Function  TreatAsAtomicUnit=on
  flag : Outport
  wires:
  eular/1 -> manoeuvrable check/2(eular)
  manoeuvrable check/1(flag) -> flag/1
  fn/1 -> manoeuvrable check/1(fn)

== system main_RI_LIEKF_GNSSOutrage/State estimation/distribute CF/AHRS/Init_Q0/Horizontal_attitude/Deal with zero ==
  In1 : Inport
  Add5 : Sum
  Constant1 : Constant  Value=1e-6  OutDataTypeStr=single
  Out1 : Outport
  wires:
  Constant1/1 -> Add5/2
  In1/1 -> Add5/1
  Add5/1 -> Out1/1

== system main_RI_LIEKF_GNSSOutrage/State estimation/distribute CF/Translation_estimate/Rxy_Horizontal_estimation/Rxy_kalman filter2/Vxy kalman filter ==
  Z : Inport
  F : Inport  Port=2
  G : Inport  Port=3
  H : Inport  Port=4
  Q : Inport  Port=5
  R : Inport  Port=6
  X : Inport  Port=7
  P0 : Inport  Port=8
  Enable : Inport  Port=9
  Add1 : Sum
  Delay : Delay  DelayLength=1  InitialConditionSource=Input port
      settings: InputPortMap=u0,p4
  Gain4 : Gain  Gain=0.5
  Math Function : Math  Operator=transpose  SignedPower=on
  kalman : Subsystem
  XOut : Outport
  wires:
  P0/1 -> Delay/2
  Gain4/1 -> Delay/1
  Delay/1 -> kalman/7(P)
  Add1/1 -> Gain4/1
  Math Function/1 -> Add1/2
  Z/1 -> kalman/1(Z)
  F/1 -> kalman/2(F)
  G/1 -> kalman/3(G)
  H/1 -> kalman/4(H)
  Q/1 -> kalman/5(Q)
  R/1 -> kalman/6(R)
  X/1 -> kalman/8(X)
  kalman/1(POut) -> Math Function/1, Add1/1
  kalman/2(XOut) -> XOut/1
  Enable/1 -> kalman/9(Enable)

== system main_RI_LIEKF_GNSSOutrage/State estimation/distribute CF/Translation_estimate/V_Horizontal_estimation/Rxy_kalman filter1/Vxy kalman filter ==
  Z : Inport
  F : Inport  Port=2
  G : Inport  Port=3
  H : Inport  Port=4
  Q : Inport  Port=5
  R : Inport  Port=6
  X : Inport  Port=7
  P0 : Inport  Port=8
  Enable : Inport  Port=9
  Add1 : Sum
  Delay : Delay  DelayLength=1  InitialConditionSource=Input port
      settings: InputPortMap=u0,p4
  Gain4 : Gain  Gain=0.5
  Math Function : Math  Operator=transpose  SignedPower=on
  kalman : Subsystem
  XOut : Outport
  wires:
  Enable/1 -> kalman/9(Enable)
  kalman/2(XOut) -> XOut/1
  kalman/1(POut) -> Add1/1, Math Function/1
  X/1 -> kalman/8(X)
  R/1 -> kalman/6(R)
  Q/1 -> kalman/5(Q)
  H/1 -> kalman/4(H)
  G/1 -> kalman/3(G)
  F/1 -> kalman/2(F)
  Z/1 -> kalman/1(Z)
  Math Function/1 -> Add1/2
  Add1/1 -> Gain4/1
  Delay/1 -> kalman/7(P)
  Gain4/1 -> Delay/1
  P0/1 -> Delay/2

== system main_RI_LIEKF_GNSSOutrage/State estimation/distribute CF/distribute CF/AHRS1/Bus_Constructor/Euler_Angle ==
  att_quat : Inport
  Demux : Demux  Outputs=3
  Quaternion To Euler : FMT_Model_Lib/Quaternion/Quaternion To Euler
  phi_rad : Outport
  theta_rad : Outport  Port=2
  psi_rad : Outport  Port=3
  wires:
  Demux/1 -> phi_rad/1
  Demux/2 -> theta_rad/1
  Demux/3 -> psi_rad/1
  att_quat/1 -> Quaternion To Euler/1
  Quaternion To Euler/1 -> Demux/1

== system main_RI_LIEKF_GNSSOutrage/State estimation/distribute CF/distribute CF/AHRS1/Correct/Attitude_Correction ==
  Sensor_Data : Inport
  Rotation_Data : Inport  Port=2
  standstill : Inport  Port=3
  Attitude_Correct : Subsystem
  Bus Selector2 : BusSelector  OutputSignals=M_BO
  Mag_Correct : Subsystem
  Multiply : Product  Multiplication=Matrix(*)
  Sum : Sum  Inputs=|++
  att_B_correction : Outport
  wires:
  standstill/1 -> Mag_Correct/3(standstill)
  Sensor_Data/1 -> Attitude_Correct/2(Sensor_Data), Mag_Correct/2(Sensor_Data)
  Attitude_Correct/1(att_corr_O) -> Sum/1  "att_corr_O"
  Mag_Correct/1(mag_corr_O) -> Sum/2  "mag_corr_O"
  Multiply/1 -> att_B_correction/1
  Rotation_Data/1 -> Mag_Correct/1(Rotation_Data), Bus Selector2/1, Attitude_Correct/1(Rotation_Data)
  Sum/1 -> Multiply/2
  Bus Selector2/1 -> Multiply/1  "<M_BO>"

== system main_RI_LIEKF_GNSSOutrage/State estimation/distribute CF/distribute CF/AHRS1/Correct/Gyro_Bias_Correction ==
  att_B_correction : Inport
  IMU_Data : Inport  Port=2
  Abs : Abs  SaturateOnIntegerOverflow=off
  Bus Selector : BusSelector  OutputSignals=acc_B_mPs2
  Compare To Constant : simulink/Logic and Bit Operations/Compare To Constant  relop=<=  const=1  OutDataTypeStr=boolean
  Constant : Constant  Value=INS_CONST.g  OutDataTypeStr=single
  Data Type Conversion : DataTypeConversion  OutDataTypeStr=single  SaturateOnIntegerOverflow=off  RndMeth=Floor
  Gain1 : Gain  Gain=INS_PARAM.BIAS_G_GAIN
  MX Product1 : Product  RndMeth=Simplest
  Saturation2 : Saturate  UpperLimit=0.1/180*pi  LowerLimit=-0.1/180*pi
  Second Order LPF : FMT_Model_Lib/Filter/Second Order LPF  fc=5  zeta=0.707
  Subtract : Sum  Inputs=+-
  Vector Modulus : FMT_Model_Lib/Math/Vector Modulus
  bias_g_B_correction : Outport
  wires:
  IMU_Data/1 -> Bus Selector/1
  Saturation2/1 -> bias_g_B_correction/1  "bias_g_correction"
  Compare To Constant/1 -> Data Type Conversion/1
  Bus Selector/1 -> Vector Modulus/1  "<acc_B_mPs2>"
  MX Product1/1 -> Second Order LPF/1
  att_B_correction/1 -> MX Product1/1
  Vector Modulus/1 -> Subtract/1
  Gain1/1 -> Saturation2/1
  Constant/1 -> Subtract/2
  Subtract/1 -> Abs/1
  Abs/1 -> Compare To Constant/1
  Data Type Conversion/1 -> MX Product1/2
  Second Order LPF/1 -> Gain1/1

== system main_RI_LIEKF_GNSSOutrage/State estimation/distribute CF/distribute CF/AHRS1/Update/Attitude_Update ==
  att_reset : Inport
  quat_0 : Inport  Port=2
  att_B_correction : Inport  Port=3
  Constant : Constant  Value=0  OutDataTypeStr=single
  Discrete-Time Integrator : DiscreteIntegrator  ExternalReset=level  InitialConditionSource=external  SampleTime=-1  ICPrevOutput=DiscIntNeverNeededParam  ICPrevScaledInput=DiscIntNeverNeededParam
  Gain2 : Gain  Gain=0.5  OutMin=-450*pi/180  OutMax=450*pi/180  RndMeth=Simplest
  Mux1 : Mux  Inputs=2
  Quaternion Multiply : FMT_Model_Lib/Quaternion/Quaternion Multiply
  Quaternion Normalize : FMT_Model_Lib/Quaternion/Quaternion Normalize
  Quaternion To DCM : FMT_Model_Lib/Quaternion/Quaternion To DCM
  Transpose : Math  Operator=transpose  SignedPower=on
  att_quat : Outport
  DCM_OB : Outport  Port=2
  wires:
  att_reset/1 -> Discrete-Time Integrator/2
  quat_0/1 -> Discrete-Time Integrator/3
  Gain2/1 -> Discrete-Time Integrator/1
  Quaternion Multiply/1 -> Gain2/1
  att_B_correction/1 -> Mux1/2
  Mux1/1 -> Quaternion Multiply/2
  Constant/1 -> Mux1/1
  Quaternion Normalize/1 -> Quaternion To DCM/1, Quaternion Multiply/1, att_quat/1
  Discrete-Time Integrator/1 -> Quaternion Normalize/1
  Quaternion To DCM/1 -> Transpose/1
  Transpose/1 -> DCM_OB/1

== system main_RI_LIEKF_GNSSOutrage/State estimation/distribute CF/distribute CF/AHRS1/Update/Gyro_Bias_Update ==
  bias_g_correction : Inport
  gyr_B_radPs : Inport  Port=2
  Discrete-Time Integrator2 : DiscreteIntegrator  SampleTime=-1  LimitOutput=on  UpperSaturationLimit=45/180*pi  LowerSaturationLimit=-45/180*pi  ICPrevOutput=DiscIntNeverNeededParam  ICPrevScaledInput=DiscIntNeverNeededParam
  Sum1 : Sum  Inputs=++|
  gyr_B_correction : Outport
  bias_g : Outport  Port=2
  wires:
  bias_g_correction/1 -> Discrete-Time Integrator2/1
  Sum1/1 -> gyr_B_correction/1
  Discrete-Time Integrator2/1 -> Sum1/1, bias_g/1
  gyr_B_radPs/1 -> Sum1/2

== system main_RI_LIEKF_GNSSOutrage/State estimation/distribute CF/distribute CF/Bus_Constructor/Subsystem1/Subsystem ==
  psi : Inport
  Constant{,1..3} (4 alike) : Constant  Value=0  OutDataTypeStr=single
  Constant4 : Constant  OutDataTypeStr=single
  Cos : Trigonometry  Operator=cos
  Cos1 : Trigonometry  Operator=cos
  Gain : Gain  Gain=-1
  Sin : Trigonometry
  Sin1 : Trigonometry
  Vector Concatenate : Concatenate  NumInputs=3  Mode=Multidimensional array
  Vector Concatenate1 : Concatenate  NumInputs=3  Mode=Multidimensional array
  Vector Concatenate2 : Concatenate  NumInputs=3  Mode=Multidimensional array
  Vector Concatenate3 : Concatenate  NumInputs=3  Mode=Multidimensional array  ConcatenateDimension=2
  DCMz : Outport
  wires:
  Constant3/1 -> Vector Concatenate2/2
  Cos/1 -> Vector Concatenate/1
  Vector Concatenate1/1 -> Vector Concatenate3/2
  Gain/1 -> Vector Concatenate1/1
  Constant1/1 -> Vector Concatenate1/3
  Sin/1 -> Vector Concatenate/2
  psi/1 -> Cos1/1, Sin1/1, Sin/1, Cos/1
  Constant2/1 -> Vector Concatenate2/1
  Sin1/1 -> Gain/1
  Constant/1 -> Vector Concatenate/3
  Cos1/1 -> Vector Concatenate1/2
  Vector Concatenate2/1 -> Vector Concatenate3/3
  Vector Concatenate/1 -> Vector Concatenate3/1
  Constant4/1 -> Vector Concatenate2/3
  Vector Concatenate3/1 -> DCMz/1

== system main_RI_LIEKF_GNSSOutrage/State estimation/distribute CF/distribute CF/Correct/Attitude_Correction/Attitude_Correct ==
  Sensor_Data : Inport
  Rotation_Data : Inport  Port=2
  Acc_Correct : Subsystem
  Subsystem2 : Subsystem
  att_corr_O : Outport
  wires:
  Subsystem2/2(acc_meas_O_mPs2) -> Acc_Correct/2(acc_meas_O_mPs2)  "GPS-加速度估计"
  Acc_Correct/1(att_correct) -> att_corr_O/1
  Subsystem2/3(acc_est_O_mPs2) -> Acc_Correct/3(acc_est_O_mPs2)  "加计-加速度"
  Subsystem2/1(acc_meas_valid) -> Acc_Correct/1(acc_meas_valid)  "GPS状态判断"
  Sensor_Data/1 -> Subsystem2/1(Sensor_Data)
  Rotation_Data/1 -> Subsystem2/2(Rotation_Data)

== system main_RI_LIEKF_GNSSOutrage/State estimation/distribute CF/distribute CF/Correct/Attitude_Correction/Mag_Correct ==
  Rotation_Data : Inport
  Sensor_Data : Inport  Port=2
  Bus Selector1 : BusSelector  OutputSignals=MAGN_Data.mag_norm_B,MAGN_Data.mag_quality
  Bus Selector4 : BusSelector  OutputSignals=M_OB
  MX Product3 : Product  Inputs=3  RndMeth=Simplest
  MX Product4 : Product  Multiplication=Matrix(*)  RndMeth=Simplest
  Relay1 : Relay  OnSwitchValue=0.3  OffSwitchValue=0.2
  Selector4 : Selector  NumberOfDimensions=2  InputPortWidth=3  IndexOptions=Index vector (dialog),Index vector (dialog)  Indices=[2],[1 2 3]  OutputSizes=1,1
  Z axis : Constant  Value=[0 0 1]  OutDataTypeStr=single
  mag_correct_gain : Gain  Gain=MAG_GAIN  OutDataTypeStr=Inherit: Same as input
  mag_corr_O : Outport  VectorParamsAs1DForOutWhenUnconnected=off
  wires:
  Bus Selector4/1 -> Selector4/1  "<M_OB>"
  Rotation_Data/1 -> Bus Selector4/1
  Bus Selector1/2 -> Relay1/1  "<mag_quality>"
  Sensor_Data/1 -> Bus Selector1/1
  mag_correct_gain/1 -> MX Product3/2
  MX Product4/1 -> mag_correct_gain/1  "my_O"
  Selector4/1 -> MX Product4/1
  Relay1/1 -> MX Product3/3  "mag_enable"
  MX Product3/1 -> mag_corr_O/1
  Bus Selector1/1 -> MX Product4/2  "<mag_norm_B>"
  Z axis/1 -> MX Product3/1

== system main_RI_LIEKF_GNSSOutrage/State estimation/distribute CF/distribute CF/Correct/Subsystem2/norm ==
  In1 : Inport
  Sqrt : Sqrt
  Square : Math  Operator=square  SignedPower=on
  Sum of Elements : Sum  Inputs=+
  Out1 : Outport
  wires:
  Sum of Elements/1 -> Sqrt/1
  Square/1 -> Sum of Elements/1
  Sqrt/1 -> Out1/1
  In1/1 -> Square/1

== system main_RI_LIEKF_GNSSOutrage/State estimation/distribute CF/distribute CF/Correct/Subsystem2/低通滤波 ==
  u : Inport
  Constant : Constant  Value=0
  Discrete-Time Integrator : DiscreteIntegrator  ExternalReset=level  SampleTime=-1  ICPrevOutput=DiscIntNeverNeededParam  ICPrevScaledInput=DiscIntNeverNeededParam
  Discrete-Time Integrator1 : DiscreteIntegrator  ExternalReset=level  InitialConditionSource=external  SampleTime=-1  ICPrevOutput=DiscIntNeverNeededParam  ICPrevScaledInput=DiscIntNeverNeededParam
  Gain : Gain  Gain=(2*pi*fc)^2
  Gain1 : Gain  Gain=2*zeta*(2*pi*fc)
  Sum : Sum  Inputs=|+-
  Sum1 : Sum  Inputs=|+-
  y : Outport
  wires:
  Sum/1 -> Gain/1
  Discrete-Time Integrator1/1 -> y/1, Sum/2
  Discrete-Time Integrator/1 -> Gain1/1, Discrete-Time Integrator1/1
  Sum1/1 -> Discrete-Time Integrator/1
  Constant/1 -> Discrete-Time Integrator1/2, Discrete-Time Integrator/2
  u/1 -> Discrete-Time Integrator1/3, Sum/1
  Gain1/1 -> Sum1/2
  Gain/1 -> Sum1/1

== system main_RI_LIEKF_GNSSOutrage/State estimation/distribute CF/distribute CF/Translation_estimate/Rxy_Horizontal_estimation/Integrator_R_Horizontal ==
  Vn : Inport
  dR : Inport  Port=2
  Sensor_data2 : Inport  Port=3
  Cbn : Inport  Port=4
  Add : Sum
  Bus Selector : BusSelector  OutputSignals=QGC_sensor_reinit,GPS_Data.pos_N_gps,GPS_Data.pos_E_gps
  Constant : Constant  Value=[-0.45;0;0]  OutDataTypeStr=single
  Delay : Delay  DelayLength=1  InitialConditionSource=Input port  ExternalReset=Rising
      settings: InputPortMap=u0,r5,p4
  Gain : Gain  Gain=0.1
  Gain2 : Gain  Gain=dt  SaturateOnIntegerOverflow=on  OutDataTypeStr=Inherit: Same as input  ParamDataTypeStr=Inherit: Same as input
  Mux : Mux  Inputs=2
  Product : Product  Multiplication=Matrix(*)
  Selector : Selector  InputPortWidth=3  IndexOptions=Index vector (dialog)  Indices=[1 2]  OutputSizes=1
  Sum : Sum  Inputs=|++-
  R_n&e : Outport
  R_n&eL : Outport  Port=2
  wires:
  dR/1 -> Gain/1
  Vn/1 -> Gain2/1
  Gain2/1 -> Sum/1
  Sensor_data2/1 -> Bus Selector/1
  Bus Selector/1 -> Delay/2  "<QGC_sensor_reinit>"
  Bus Selector/2 -> Mux/1  "<pos_N_gps>"
  Bus Selector/3 -> Mux/2  "<pos_E_gps>"
  Mux/1 -> Delay/3
  Delay/1 -> Sum/2
  Gain/1 -> Sum/3
  Constant/1 -> Product/2
  Product/1 -> Selector/1
  Cbn/1 -> Product/1
  Sum/1 -> Add/1, R_n&e/1, Delay/1
  Selector/1 -> Add/2
  Add/1 -> R_n&eL/1

== system main_RI_LIEKF_GNSSOutrage/State estimation/distribute CF/distribute CF/Translation_estimate/Rxy_Horizontal_estimation/Rxy_kalman filter2 ==
  X : Inport
  Z : Inport  Port=2
  Enable : Inport  Port=3
  Constant : Constant  Value=F  OutDataTypeStr=single
  Constant1 : Constant  Value=Q  OutDataTypeStr=single
  Constant2 : Constant  Value=R  OutDataTypeStr=single
  Constant3 : Constant  Value=P0  OutDataTypeStr=single
  Constant4 : Constant  Value=H  OutDataTypeStr=single
  Vxy kalman filter : Subsystem  TreatAsAtomicUnit=on
  XOut : Outport
  wires:
  Enable/1 -> Vxy kalman filter/9(Enable)
  Vxy kalman filter/1(XOut) -> XOut/1
  Constant1/1 -> Vxy kalman filter/5(Q)
  Constant4/1 -> Vxy kalman filter/4(H)
  Constant2/1 -> Vxy kalman filter/6(R)
  Constant3/1 -> Vxy kalman filter/8(P0)
  Z/1 -> Vxy kalman filter/1(Z)
  Constant/1 -> Vxy kalman filter/3(G), Vxy kalman filter/2(F)
  X/1 -> Vxy kalman filter/7(X)

== system main_RI_LIEKF_GNSSOutrage/State estimation/distribute CF/distribute CF/Translation_estimate/Rxy_Horizontal_estimation/Subsystem ==
  Detect Change1 : simulink/Logic and Bit Operations/Detect Change  vinit=0  InputProcessing=Columns as channels (frame based)  OutDataTypeStr=boolean
  From Workspace1 : FromWorkspace  VariableName=[All.t',All.lat]
  flag : Outport
  wires:
  Detect Change1/1 -> flag/1
  From Workspace1/1 -> Detect Change1/1  "lat"
